simulink model "foerderband_sil"  (R2025b)
settings: Solver=ode23tb  StartTime=0.0  StopTime=60  FixedStep=0.005  MinStep=0.01  RelTol=1e-3
InitFcn:
  | wrapperPIDController(0,0,true,true)
undefined symbols (not defined in the file or in its folder): wrapperPIDController
settings Model: Creator=tczuest  LastModifiedBy=JumpStart
settings SolverCC: AlgebraicLoopSolver=TrustRegion
settings DebuggingCC: UnconnectedInputMsg=warning  UnconnectedOutputMsg=warning  UnconnectedLineMsg=warning
settings ModelReferenceCC: EnableRefExpFcnMdlSchedulingChecks=on
settings RTWCC: GPUComputeCapability=3.5  DLArmComputeVersion=19.05

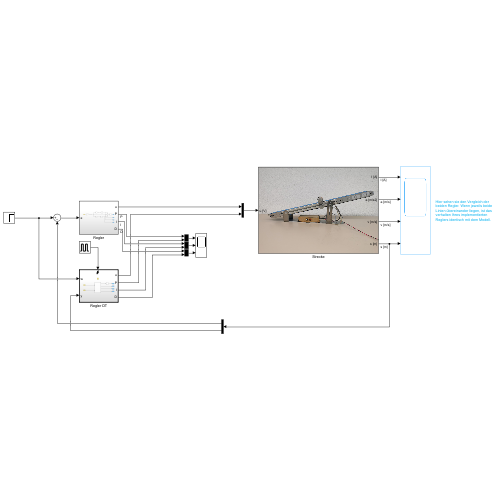
[thumbnail: Simulink's stored preview of the top-level diagram]
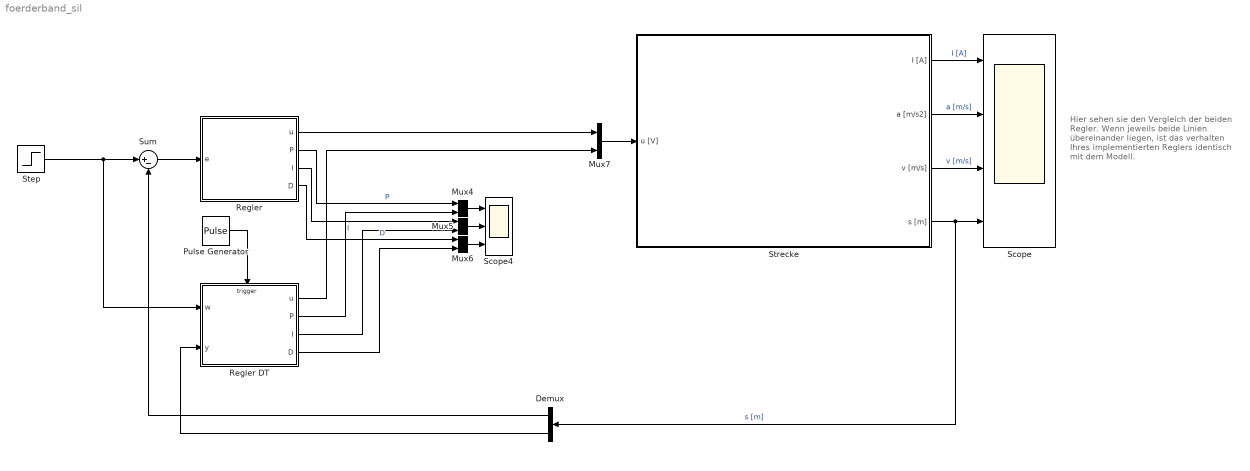
== system foerderband_sil ==
  note: Hier sehen sie den Vergleich der beiden Regler. Wenn jeweils beide Linien übereinander liegen, ist das verhalten Ihres implementierten Reglers identisch mit dem Modell.
  Demux : Demux  Outputs=2
  Mux{4..7} (4 alike) : Mux  Inputs=2
  Pulse Generator : DiscretePulseGenerator  PulseType=Time based  Period=0.01  PulseWidth=50
  Regler : Subsystem
  Regler DT : Subsystem  InitFcn=wrapperPIDController(0, 0, true, true)
  Scope : Scope  NumInputPorts=4
      settings: ActiveDisplayString=4  ActiveDisplayYMinimum=-0.055625178302072191  ActiveDisplayYMaximum=0.50062660471864984
  Scope4 : Scope  NumInputPorts=3
      settings: ActiveDisplayString=3  ActiveDisplayYMinimum=-1  ActiveDisplayYMaximum=1  DataLoggingVariableName=ScopeData2
  Step : Step  Time=15  After=0.415  SampleTime=0
  Strecke : Subsystem
      mask Display: image('$imagefile'); % Use "Edit Image" on toolstrip to change.
  Sum : Sum  Inputs=|+-
  wires:
  Step/1 -> Regler DT/1(w), Sum/1
  Strecke/1(I [A]) -> Scope/1  "I [A]"
  Strecke/2(a [m/s2]) -> Scope/2  "a [m/s]"
  Strecke/3(v [m/s]) -> Scope/3  "v [m/s]"
  Strecke/4(s [m]) -> Scope/4, Demux/1  "s [m]"
  Regler/1(u) -> Mux7/1
  Regler/2(P) -> Mux4/1  "P"
  Regler/3(I) -> Mux5/1  "I"
  Regler/4(D) -> Mux6/1  "D"
  Regler DT/1(u) -> Mux7/2
  Regler DT/2(P) -> Mux4/2
  Regler DT/3(I) -> Mux5/2
  Regler DT/4(D) -> Mux6/2
  Pulse Generator/1 -> Regler DT/Trigger
  Mux4/1 -> Scope4/1
  Mux5/1 -> Scope4/2
  Mux6/1 -> Scope4/3
  Sum/1 -> Regler/1(e)
  Demux/1 -> Sum/2
  Demux/2 -> Regler DT/2(y)
  Mux7/1 -> Strecke/1(u [V])

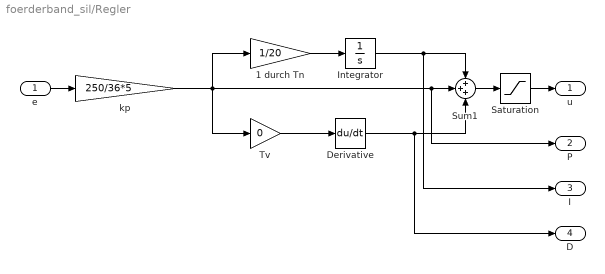
== system foerderband_sil/Regler ==
  e : Inport
  1 durch Tn : Gain  Gain=1/20
  Derivative : Derivative
  Integrator : Integrator  LimitOutput=on  UpperSaturationLimit=5  LowerSaturationLimit=-5
  Saturation : Saturate  UpperLimit=5  LowerLimit=-5
  Sum1 : Sum  Inputs=+++
  Tv : Gain  Gain=0
  kp : Gain  Gain=250/36*5
  u : Outport
  P : Outport  Port=2
  I : Outport  Port=3
  D : Outport  Port=4
  wires:
  e/1 -> kp/1
  1 durch Tn/1 -> Integrator/1
  kp/1 -> Tv/1, 1 durch Tn/1, P/1, Sum1/2
  Integrator/1 -> I/1, Sum1/1
  Tv/1 -> Derivative/1
  Derivative/1 -> D/1, Sum1/3
  Sum1/1 -> Saturation/1
  Saturation/1 -> u/1

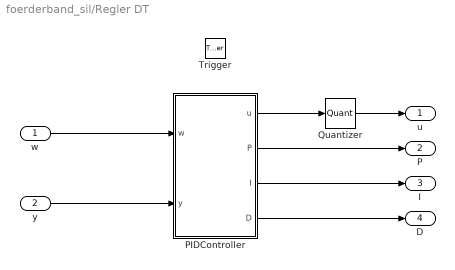
== system foerderband_sil/Regler DT ==
  w : Inport
  y : Inport  Port=2
  Trigger : TriggerPort  VariantControl=(inherit)
  PIDController : MATLAB Function  TreatAsAtomicUnit=on
  Quantizer : Quantizer  QuantizationInterval=5/1023
  u : Outport
  P : Outport  Port=2
  I : Outport  Port=3
  D : Outport  Port=4
  wires:
  w/1 -> PIDController/1(w)
  PIDController/1(u) -> Quantizer/1
  PIDController/2(P) -> P/1
  PIDController/3(I) -> I/1
  PIDController/4(D) -> D/1
  y/1 -> PIDController/2(y)
  Quantizer/1 -> u/1

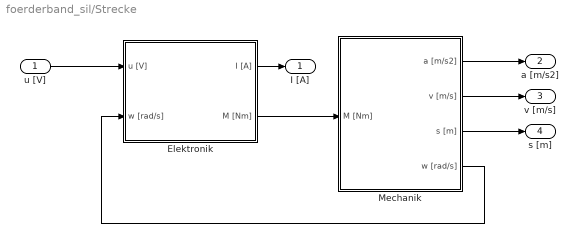
== system foerderband_sil/Strecke ==
  u [V] : Inport
  Elektronik : Subsystem
  Mechanik : Subsystem
  I [A] : Outport
  a [m/s2] : Outport  Port=2
  v [m/s] : Outport  Port=3
  s [m] : Outport  Port=4
  wires:
  Mechanik/1(a [m/s2]) -> a [m/s2]/1
  Mechanik/2(v [m/s]) -> v [m/s]/1
  Mechanik/3(s [m]) -> s [m]/1
  Elektronik/2(M [Nm]) -> Mechanik/1(M [Nm])
  Elektronik/1(I [A]) -> I [A]/1
  Mechanik/4(w [rad/s]) -> Elektronik/2(w [rad/s])
  u [V]/1 -> Elektronik/1(u [V])

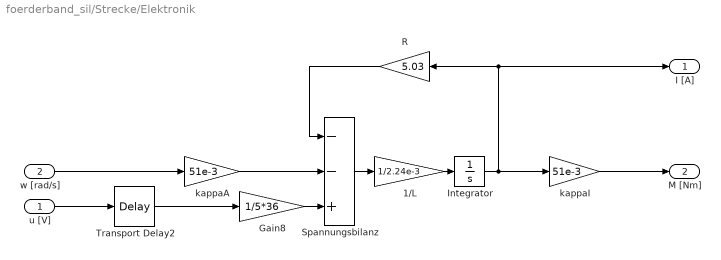
== system foerderband_sil/Strecke/Elektronik ==
  u [V] : Inport
  w [rad/s] : Inport  Port=2
  1/L : Gain  Gain=1/2.24e-3
  Gain8 : Gain  Gain=1/5*36
  Integrator : Integrator  LimitOutput=on  UpperSaturationLimit=10  LowerSaturationLimit=-10
  R : Gain  Gain=5.03
  Spannungsbilanz : Sum  Inputs=--+
  Transport Delay2 : TransportDelay  DelayTime=0.1
  kappaA : Gain  Gain=51e-3
  kappaI : Gain  Gain=51e-3
  I [A] : Outport
  M [Nm] : Outport  Port=2
  wires:
  w [rad/s]/1 -> kappaA/1
  u [V]/1 -> Transport Delay2/1
  kappaA/1 -> Spannungsbilanz/2
  R/1 -> Spannungsbilanz/1
  Spannungsbilanz/1 -> 1/L/1
  Integrator/1 -> kappaI/1, I [A]/1, R/1
  1/L/1 -> Integrator/1
  kappaI/1 -> M [Nm]/1
  Gain8/1 -> Spannungsbilanz/3
  Transport Delay2/1 -> Gain8/1

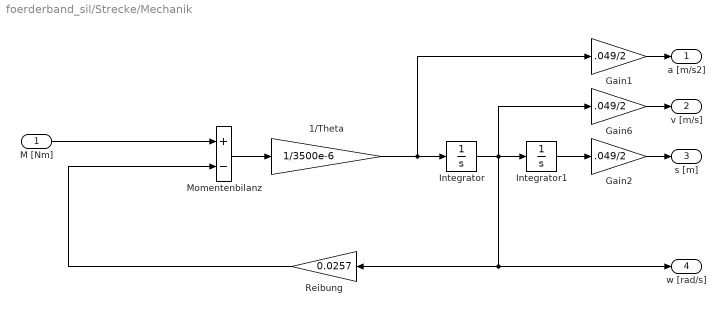
== system foerderband_sil/Strecke/Mechanik ==
  M [Nm] : Inport
  1/Theta : Gain  Gain=1/3500e-6
  Gain1 : Gain  Gain=.049/2
  Gain2 : Gain  Gain=.049/2
  Gain6 : Gain  Gain=.049/2
  Integrator : Integrator
  Integrator1 : Integrator
  Momentenbilanz : Sum  Inputs=+-
  Reibung : Gain  Gain=0.0257
  a [m/s2] : Outport
  v [m/s] : Outport  Port=2
  s [m] : Outport  Port=3
  w [rad/s] : Outport  Port=4
  wires:
  Integrator1/1 -> Gain2/1
  M [Nm]/1 -> Momentenbilanz/1
  Integrator/1 -> w [rad/s]/1, Reibung/1, Gain6/1, Integrator1/1
  Momentenbilanz/1 -> 1/Theta/1
  Reibung/1 -> Momentenbilanz/2
  Gain6/1 -> v [m/s]/1
  Gain1/1 -> a [m/s2]/1
  Gain2/1 -> s [m]/1
  1/Theta/1 -> Gain1/1, Integrator/1

== matlab function foerderband_sil/Regler DT/PIDController ==
  data: w input; u output double size=1; P output double size=1; I output double size=1; D output double size=1; y input
function [u, P, I, D] = Controller(w, y)
%#codegen
    
    coder.extrinsic('wrapperPIDController');
    [u, P, I, D] = wrapperPIDController(w, y, true);
